simulink model "Dyn_PointMass_r2019b"  (R2022b)
settings: Solver=ode4  StartTime=0.0  StopTime=simInit.TSIM  FixedStep=simInit.dt  MaxStep=simInit.dt  RelTol=1e-3
InitFcn:
  | close all
undefined symbols (not defined in the file): constr, DE2019, DiscIntNeverNeededParam, ENVMT, params, simInit
libraries: simulink x15, simulink_extras x2
(part 2 of 2)

== matlab function Dyn_PointMass_r2019b/AirborneSystem/AeroAndPropForces/Aero_prop ==
  data: F_p_B output; airdata input; DE2019 parameter; delta_t input; F_a_B output; cl_w input; cd_w input; cl_e input; cd_e input; cl_r input; cd_r input; ENVMT parameter
% Copyright 2020 Delft University of Technology
%
% Licensed under the Apache License, Version 2.0 (the "License");
% you may not use this file except in compliance with the License.
% You may obtain a copy of the License at
%
%      http://www.apache.org/licenses/LICENSE-2.0
%
% Unless required by applicable law or agreed to in writing, software
% distributed under the License is distributed on an "AS IS" BASIS,
% WITHOUT WARRANTIES OR CONDITIONS OF ANY KIND, either express or implied.
% See the License for the specific language governing permissions and
% limitations under the License.

function [F_p_B,F_a_B] = simpleAero(airdata, DE2019, delta_t,cl_w,cd_w,cl_e,cd_e,cl_r,cd_r, ENVMT)
%simpleAero - Calculate aerodynamic and propulsive forces
%
% Syntax:  [F_p_B,F_a_B] = simpleAero(airdata, aircraft_struct, delta_t,cl_w,cd_w,cl_e,cd_e,cl_r,cd_r)
%
% Inputs:
%    airdata - Wind speed, angle of attack and side slip angle
%    DE2019 - Aircraft characteristics data structure
%    delta_t - Thrust force
%    cl_w - Lift coefficient wing
%    cd_w - Drag coefficient wing
%    cl_e - Lift coefficient elevator
%    cd_e - Drag coefficient elevator
%    cl_r - Lift coefficient rudder
%    cd_r - Drag coefficient rudder
%
% Outputs:
%    F_p_B  - Propulsive forces in body reference frame
%    F_a_B  - Total aircraft aerodynamic forces in body reference frame
%   
% Example: 
%    [F_p_B,F_a_B] = simpleAero(airdata, DE2019, delta_t,cl_w,cd_w,cl_e,cd_e,cl_r,cd_r)
%
% Other m-files required: none
% Subfunctions: none
% MAT-files required: none
%
% Author: Dylan Eijkelhof, M.Sc.
% Delft University of Technology
% email address: d.eijkelhof@tudelft.nl  
% December 2019; Last revision: 30-September-2019

%------------- BEGIN CODE --------------    
    F_a_B = zeros(3,1);
    F_p_B = zeros(3,1);

    Va = airdata(1);
    alpha = airdata(2);
    beta = airdata(3);    
    Vinf = [Va*cos(alpha)*cos(beta), Va*sin(beta), Va*sin(alpha)*cos(beta)];

    q = 0.5*ENVMT.rhos*Vinf(1)^2;
    
    %% Main Wing
    F_L_main = -cl_w*q*DE2019.S_ref;
    F_D_main = cd_w*q*DE2019.S_ref;
    
    F_x_mw = -F_D_main*cos(alpha) - F_L_main*sin(alpha);
    F_z_mw = F_L_main*cos(alpha);

    %% Elevator
    F_L_el = -cl_e*q*DE2019.S_el;
    F_D_el = -cd_e*q*DE2019.S_el;
    
    F_x_el = F_D_el*cos(alpha)*cos(beta) - F_L_el*sin(alpha)*cos(beta);
    F_z_el = F_L_el*cos(alpha);
   
    %% Rudder
    F_L_vs = 2*cl_r*q*DE2019.S_vs;
    F_D_vs = -2*cd_r*q*DE2019.S_vs;

    F_x_vs = F_D_vs*cos(alpha)*cos(beta);
    F_y_vs = -F_L_vs*cos(beta);
    
    %% Sum of forces
    F_a_B = [F_x_mw+F_x_el+F_x_vs;F_y_vs; F_z_mw+F_z_el];
    
    %% Motor
%     Vd = airdata(1) + delta_t * ( DE2019.k_motor - airdata(1) );
%     Fp_x = 0.5 * 1.225 * DE2019.S_prop * DE2019.C_prop * Vd * (Vd-airdata(1));
    %% No motor, direct feed through
    F_p_B = [delta_t;0;0];
%------------- END CODE -------------- 
end
%

== matlab function Dyn_PointMass_r2019b/RequirementModelsAndLogging/MATLAB Function ==
  data: time input; eul input; stop_flag output; eul_old input
% Copyright 2021 Delft University of Technology
%
% Licensed under the Apache License, Version 2.0 (the "License");
% you may not use this file except in compliance with the License.
% You may obtain a copy of the License at
%
%      http://www.apache.org/licenses/LICENSE-2.0
%
% Unless required by applicable law or agreed to in writing, software
% distributed under the License is distributed on an "AS IS" BASIS,
% WITHOUT WARRANTIES OR CONDITIONS OF ANY KIND, either express or implied.
% See the License for the specific language governing permissions and
% limitations under the License.

function stop_flag = fcn(time, eul,eul_old)
phi = eul(1);
theta = eul(2);
% psi = eul(3);

phi_old = eul_old(1);
theta_old = eul_old(2);
% psi_old = eul_old(3);

if time>40
    if ((phi>pi/2 || phi<-pi/2) && sign(phi) ~= sign(phi_old))
        stop_flag = 1;
    elseif ((theta>pi/2 || theta<-pi/2) && sign(theta) ~= sign(theta_old))
        stop_flag = 1; 
%     elseif ((psi>pi/2 || psi<-pi/2) && sign(psi) ~= sign(psi_old))
%         stop_flag = 1; 
    else
        stop_flag = 0;
    end
else
    stop_flag = 0;
end
end
